simulink model "PIXELdithering_workbench"  (R2020a)
settings: Solver=FixedStepDiscrete  StartTime=0.0  StopTime=10.0  RelTol=1e-3
model workspace (MAT data in the model file):
  led0 = 1
  test = [240 320]
libraries: simulink x55, hdlsllib x29, visionsinks x2, visionzynq_privlib x2, visionhdlutilities x1, visiongeotforms x1, dspvision x1
(part 1 of 2)
settings Model: DataTypeOverride=Off  Creator=Produktivität  LastModifiedBy=Anwender
settings OptimizationCC: BlockReduction=off  ConditionallyExecuteInputs=off  DefaultParameterBehavior=Inlined
settings DebuggingCC: AlgebraicLoopMsg=error  SingleTaskRateTransMsg=error
settings HardwareCC: ProdBitPerPointer=32  ProdBitPerSizeT=32  ProdBitPerPtrDiffT=32  ProdLargestAtomicFloat=None  ProdIntDivRoundTo=Undefined  ProdEndianess=Unspecified  ProdWordSize=32  ProdHWDeviceType=ASIC/FPGA->ASIC/FPGA  TargetBitPerPointer=64  TargetBitPerSizeT=64  TargetBitPerPtrDiffT=64  TargetLongLongMode=on  TargetIntDivRoundTo=Zero  TargetEndianess=LittleEndian  TargetWordSize=64  TargetHWDeviceType=Custom Processor->MATLAB Host Computer  ProdEqTarget=off

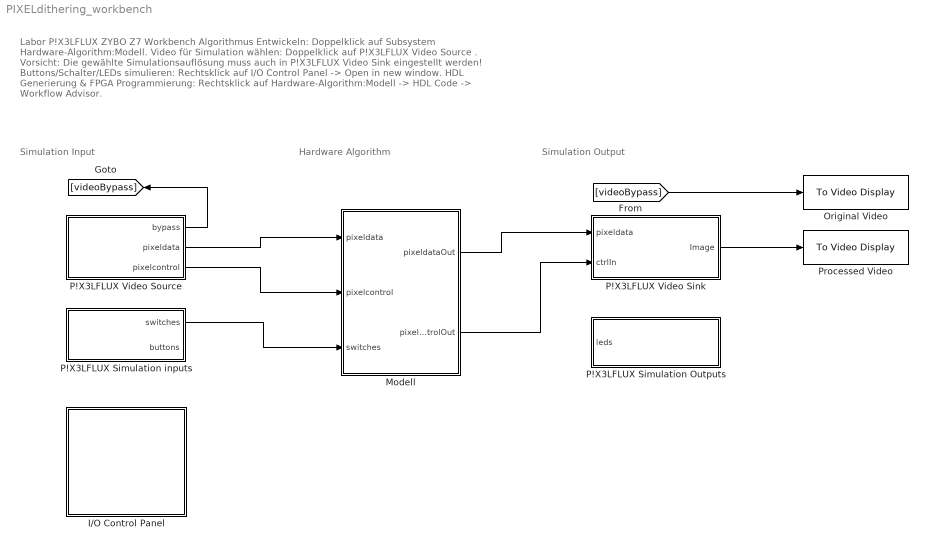
== system PIXELdithering_workbench ==
  note: Labor P!X3LFLUX
      | ZYBO Z7 Workbench
      |
      | Algorithmus Entwickeln: Doppelklick auf Subsystem Hardware-Algorithm:Modell.
      | Video für Simulation wählen: Doppelklick auf P!X3LFLUX Video Source . Vorsicht: Die gewählte Simulationsauflösung muss auch in P!X3LFLUX Video Sink eingestellt werden!
      | Buttons/Schalter/LEDs simulieren: Rechtsklick auf I/O Control Panel -> Open in new window.
      | HDL Generierung & FPGA Programmierung: Rechtsklick auf Hardware-Algorithm:Modell -> HDL Code -> Workflow Advisor.
  note: Hardware Algorithm
  note: Simulation Output
  note: Simulation Input
  I/O Control Panel : Subsystem
  Modell : Subsystem  TreatAsAtomicUnit=on
  Original Video : visionsinks/To Video Display  windowSizeMode=Normal  openAtMdlStart=on  fullScreen=off  videoWindowX=1  videoWindowY=33  saveWindowSize=off  videoWindowWidth=1916  videoWindowHeight=1006  inputColorFormat=RGB  inputType=Obsolete  imagePorts=One multidimensional signal  OutputDevice=On-screen video monitor  dataOrg=Column-major  isWindowOpen=off
  P!X3LFLUX Simulation Outputs : Subsystem
  P!X3LFLUX Simulation inputs : Subsystem  mask{buttonsMode=manual, btnFileName=mlabtest.xlsx, switchesMode=manual, swFileName=mlabtest.xlsx}
      mask prompts: buttonsMode "Buttons simulation mode:"; btnFileName "Excel filename:"; switchesMode "Switches simulation mode:"; swFileName "Excel filename:"
      mask TypeOptions buttonsMode: buttons variant choice/LabelModeActiveChoice
      mask TypeOptions btnFileName: excel reader buttons/FileName
      mask TypeOptions switchesMode: switches variant choice/LabelModeActiveChoice
      mask TypeOptions swFileName: excel reader switches/FileName
      mask DialogControl DescGroupVar Prompt: P!X3LFLUX Simulation Inputs for ZYBO Z7
      mask DialogControl DescTextVar Prompt: Dieser Block erzeugt die Simulationssignale für Knöpfe und Schalter des ZYBO Z7 Boards.
      mask DialogControl Control2 Prompt: This block generates signals for simulating the switches and buttons of the ZYBO Z7 board.
      mask DialogControl Control3 Prompt: Pick manual mode to control inputs via the I/O Control Panel
      mask DialogControl btnsContainer Prompt: Buttons simulation settings
      mask DialogControl swContainer Prompt: Switches simulation settings
  P!X3LFLUX Video Sink : Subsystem  mask{resolutionChoice=320x240}
      mask prompts: resolutionChoice "Resolution:"
      mask init:
      | resolution = get_param(gcb, 'resolutionChoice');
      | streamSinkBlk = [gcb, '/streamSink'];
      | 
      | switch resolution
      |     case '320x240'
      |         set_param(streamSinkBlk, 'FrameSize', '320x240p');
      |     case '640x480'
      |         set_param(streamSinkBlk, 'FrameSize', '640x480p');
      |     case '720x480'
      |         set_param(streamSinkBlk, 'FrameSize', '480p SDTV (720x480p)');
      |     case '1280x720'
      |         set_param(streamSinkBlk, 'FrameSize', '720p HDTV (1280x720p)');
      | end
      mask TypeOptions resolutionChoice: 320x240 | 640x480 | 720x480
      mask DialogControl DescGroupVar Prompt: P!X3LFLUX Video Sink
      mask DialogControl DescTextVar Prompt: Dieser Block wandelt einen RBG (Xilinx Encoding) Pixel Stream zurück in frames.
      mask DialogControl Control3 Prompt: This block converts a RGB (Xilinx Encoding) Pixel Stream into individual frames.
      mask DialogControl resHint Prompt: Note: Should match source resoltution!
      mask Display: image('$imagefile'); % Use "Edit Image" on toolstrip to change.
  P!X3LFLUX Video Source : Subsystem  mask{inputFilename=C:\Users\Anwender\Documents\Pixelflux_2\Boarddateien\Testdaten\360p_foggy_island.mp4, resolutionChoice=320x240}
      mask prompts: inputFilename "dspshared:FromMMFile:InputFileName"; resolutionChoice "Scaled resolution:"
      mask init:
      | resolution = get_param(gcb, 'resolutionChoice');
      | resizeBlk = [gcb, '/resizer'];
      | streamGenBlk = [gcb, '/streamGenerator'];
      | 
      | switch resolution
      |     case '320x240'
      |         set_param(streamGenBlk, 'FrameSize', '320x240p');
      |         set_param(resizeBlk, 'outRowsCols', '[240 320]');
      |     case '640x480'
      |         set_param(streamGenBlk, 'FrameSize', '640x480p');
      |         set_param(resizeBlk, 'outRowsCols', '[480 640]');
      |     case '720x480'
      |         set_param(streamGenBlk, 'FrameSize', '480p SDTV (720x480p)');
      |         set_param(resizeBlk, 'outRowsCols', '[480 720]');
      |     case '1280x720'
      |         set_param(streamGenBlk, 'FrameSize', '720p HDTV (1280x720p)');
      |         set_param(resizeBlk, 'outRowsCols', '[720 1280]');
      | end
      mask TypeOptions inputFilename: videoInput/inputFilename
      mask TypeOptions resolutionChoice: 320x240 | 640x480 | 720x480
      mask DialogControl DescGroupVar Prompt: P!X3LFLUX Lab Source
      mask DialogControl DescTextVar Prompt: Dieser Block kapselt das Einlesen eines Videofiles, Skalierung auf eine feste Auflösung sowie die Erzeugung des PixelStreams.
      mask DialogControl Control3 Prompt: This block encapsulates reading an input video file, scaling it to a fixed resolution and creating the pixel stream.
      mask DialogControl inputFilename Prompt: Input file name:
      mask DialogControl browseBtn Prompt: Browse...
      mask DialogControl browseBtn Callback:
      | [f p] = uigetfile;
      | if(f ~= 0)
      |     set_param(gcb, "inputFilename", fullfile(p, f));
      | end
      mask Display: image('$imagefile'); % Use "Edit Image" on toolstrip to change.
  Processed Video : visionsinks/To Video Display  windowSizeMode=Normal  openAtMdlStart=on  fullScreen=off  videoWindowX=1  videoWindowY=33  saveWindowSize=off  videoWindowWidth=1916  videoWindowHeight=1006  inputColorFormat=RGB  inputType=Obsolete  imagePorts=One multidimensional signal  OutputDevice=On-screen video monitor  dataOrg=Column-major  isWindowOpen=off
  wires:
  [videoBypass] -> Original Video/1
  P!X3LFLUX Video Source/1(bypass) -> [videoBypass]
  Modell/1(pixeldataOut) -> P!X3LFLUX Video Sink/1(pixeldata)
  Modell/2(pixelcontrolOut) -> P!X3LFLUX Video Sink/2(ctrlIn)
  P!X3LFLUX Video Sink/1(Image) -> Processed Video/1
  P!X3LFLUX Video Source/2(pixeldata) -> Modell/1(pixeldata)
  P!X3LFLUX Video Source/3(pixelcontrol) -> Modell/2(pixelcontrol)
  P!X3LFLUX Simulation inputs/1(switches) -> Modell/3(switches)

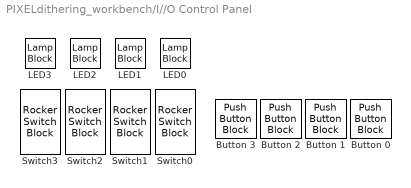
== system PIXELdithering_workbench/I//O Control Panel ==
  Button 0 : PushButtonBlock  ButtonText=0
  Button 1 : PushButtonBlock  ButtonText=1
  Button 2 : PushButtonBlock  ButtonText=2
  Button 3 : PushButtonBlock  ButtonText=3
  LED{0..3} (4 alike) : LampBlock  LabelPosition=Hide
  Switch{0..3} (4 alike) : RockerSwitchBlock  LabelPosition=Hide
      settings: Values={{'Off', 'On'}, [0 1]}

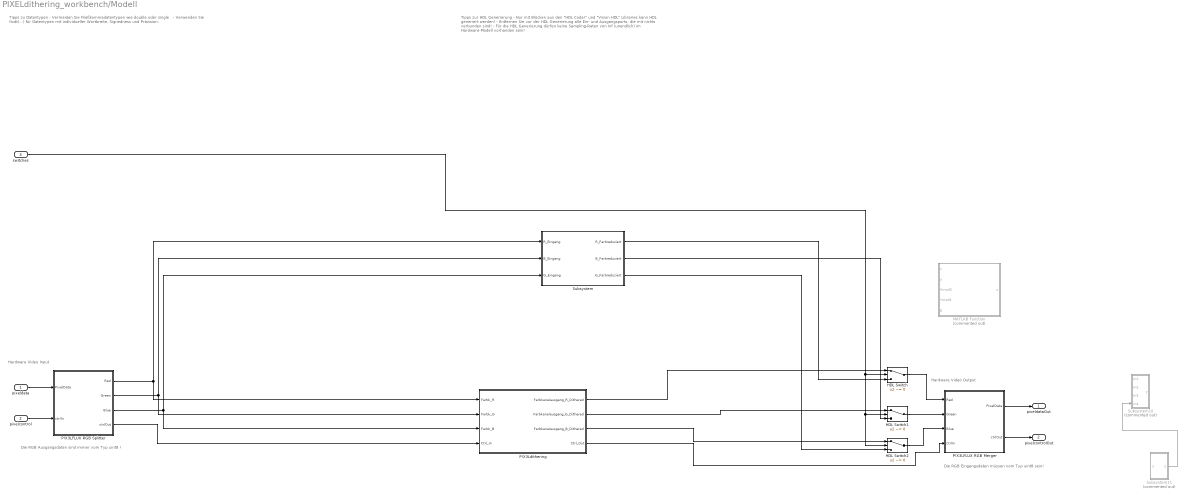
== system PIXELdithering_workbench/Modell ==
  note: Tipps zur HDL Generierung
      |
      | - Nur mit Blöcken aus den "HDL Coder" und "Vision HDL" Libraries kann HDL generiert werden!
      | - Entfernen Sie vor der HDL Generierung alle Ein- und Ausgangsports, die mit nichts verbunden sind!
      | - Für die HDL Generierung dürfen keine Sampling-Raten von Inf (unendlich) im Hardware-Modell vorhanden sein!
  note: Die RGB Ausgangsdaten sind immer vom Typ uint8 !
  note: Hardware Video Output
  note: Hardware Video Input
  note: Die RGB Eingangsdaten müssen vom Typ uint8 sein!
  note: Tipps zu Datentypen
      |
      | - Vermeiden Sie Fließkommadatentypen wie double oder single .
      | - Verwenden Sie fixdt(...) für Datentypen mit individueller Wortbreite, Signedness und Präzision.
  pixeldata : Inport  OutDataTypeStr=fixdt(0,24,0)
  pixelcontrol : Inport  Port=2  OutDataTypeStr=Bus: pixelcontrol
  switches : Inport  Port=3  OutDataTypeStr=fixdt(0,4,0)
  HDL Switch : Switch  Criteria=u2 ~= 0  Threshold=960  OutDataTypeStr=uint8
  HDL Switch1 : Switch  Criteria=u2 ~= 0  Threshold=960  OutDataTypeStr=uint8
  HDL Switch2 : Switch  Criteria=u2 ~= 0  Threshold=960  OutDataTypeStr=uint8
  MATLAB Function : MATLAB Function  Commented=on  TreatAsAtomicUnit=on
  P!X3LFLUX RGB Merger : Subsystem  Variant=on  VariantControlMode=Label  VariantControl=Choice  LabelModeActiveChoice=V_sepColor  mask{InputVersionChoice=Separate components}
      mask prompts: InputVersionChoice "Color component input mode:"
      mask init:
      | choice = get_param(gcb,'InputVersionChoice');
      | vssBlk = gcb;
      | 
      | rgbInput = find_system(gcb,...
      |     'LookUnderMasks', 'on',...
      |     'FollowLinks', 'on',...
      |     'Name', 'rgb');
      | 
      | oldVariant = get_param(gcb,'LabelModeActiveChoice');
      | if strcmp(choice,'Separate components')
      |     if ~isempty(rgbInput)
      |         delete_block([gcb, '/rgb']);
      |         add_block('built-in/Inport', [gcb, '/Red'], 'Port', '1', 'OutDataTypeStr', 'uint8', 'PortDimensions', '1');
      |         add_block('built-in/Inport', [gcb, '/Green'], 'Port', '2', 'OutDataTypeStr', 'uint8', 'PortDimensions', '1');
      |         add_block('built-in/Inport', [gcb, '/Blue'], 'Port', '3', 'OutDataTypeStr', 'uint8', 'PortDimensions', '1');
      |     end
      |     set_param(vssBlk, 'OverrideUsingVariant', 'V_sepColor');
      | else
      |     if isempty(rgbInput)
      |         delete_block([gcb, '/Red']);
      |         delete_block([gcb, '/Green']);
      |         delete_block([gcb, '/Blue']);
      |         add_block('built-in/Inport', [gcb, '/rgb'], 'Port', '1', 'OutDataTypeStr', 'uint8', 'PortDimensions', '[1 3]');
      |     end
      |     set_param(vssBlk, 'OverrideUsingVariant', 'V_vecColor');
      | end
      mask TypeOptions InputVersionChoice: Separate components | RGB vector [1x3]
      mask DialogControl DescGroupVar Prompt: P!X3LFLUX RGB Merger for Xilinx AXI4 Video Stream
      mask DialogControl DescTextVar Prompt: Dieser Block bündelt 8 Bit Farbkanäle in 24 Bit RBG (Xilinx Encoding) AXI4 Video Stream Pixeldaten. Zur HDL Generierung geeignet.
      mask DialogControl Control2 Prompt: This block packs 8 Bit color components into 24 Bit RBG (Xilinx Encoding) AXI4 Video Stream pixeldata. Compatible with HDL generation.
      mask DialogControl InputVersionChoice Tooltip: Choose between separate component ports or one [1x3] vector input
      mask Display: image('$imagefile'); % Use "Edit Image" on toolstrip to change.
  P!X3LFLUX RGB Splitter : Subsystem  Variant=on  VariantControlMode=Label  LabelModeActiveChoice=V_sepColor  mask{OutputVersionChoice=Separate components}
      mask prompts: OutputVersionChoice "Color component output mode:"
      mask init:
      | choice = get_param(gcb,'OutputVersionChoice');
      | vssBlk = gcb;
      | oldVariant = get_param(gcb,'LabelModeActiveChoice');
      | rgbOut = find_system(gcb,...
      |     'LookUnderMasks', 'on',...
      |     'FollowLinks', 'on',...
      |     'Name', 'rgb');
      | 
      | if strcmp(choice,'Separate components')
      |     if ~isempty(rgbOut)
      |         delete_block([gcb, '/rgb']);
      |         add_block('built-in/Outport', [gcb, '/Red'], 'Port', '1', 'OutDataTypeStr', 'uint8', 'PortDimensions', '1');
      |         add_block('built-in/Outport', [gcb, '/Green'], 'Port', '2', 'OutDataTypeStr', 'uint8', 'PortDimensions', '1');
      |         add_block('built-in/Outport', [gcb, '/Blue'], 'Port', '3', 'OutDataTypeStr', 'uint8', 'PortDimensions', '1');
      |     end
      |     set_param(vssBlk, 'OverrideUsingVariant', 'V_sepColor');
      | else
      |     if isempty(rgbOut)
      |         delete_block([gcb, '/Red']);
      |         delete_block([gcb, '/Green']);
      |         delete_block([gcb, '/Blue']);
      |         add_block('built-in/Outport', [gcb, '/rgb'], 'Port', '1', 'OutDataTypeStr', 'uint8', 'PortDimensions', '[1 3]');
      |     end
      |     set_param(vssBlk, 'OverrideUsingVariant', 'V_vecColor');
      | end
      mask TypeOptions OutputVersionChoice: Separate components | RGB vector [1x3]
      mask DialogControl DescGroupVar Prompt: P!X3LFLUX RGB Splitter for Xilinx AXI4 Video Stream
      mask DialogControl DescGerman Prompt: Dieser Block separiert die Farbkanäle von 24 Bit RBG (Xilinx Encoding) AXI4 Video Stream Pixeldaten.
      mask DialogControl DescEnglish Prompt: This block separates the color components of 24 Bit RBG (Xilinx Encoding) AXI4 Video Stream pixel data.
      mask Display: image('$imagefile'); % Use "Edit Image" on toolstrip to change.
  P!X3Ldithering : Subsystem
  Subsystem : Subsystem
  Subsystem10 : Subsystem  Commented=on
  Subsystem11 : Subsystem  Commented=on
  pixeldataOut : Outport  OutDataTypeStr=fixdt(0,24,0)  VectorParamsAs1DForOutWhenUnconnected=off
  pixelcontrolOut : Outport  Port=2  VectorParamsAs1DForOutWhenUnconnected=off
  wires:
  P!X3LFLUX RGB Merger/1(PixelData) -> pixeldataOut/1
  P!X3LFLUX RGB Merger/2(ctrlOut) -> pixelcontrolOut/1
  pixeldata/1 -> P!X3LFLUX RGB Splitter/1(PixelData)
  pixelcontrol/1 -> P!X3LFLUX RGB Splitter/2(ctrlIn)
  HDL Switch/1 -> P!X3LFLUX RGB Merger/1(Red)
  HDL Switch1/1 -> P!X3LFLUX RGB Merger/2(Green)
  HDL Switch2/1 -> P!X3LFLUX RGB Merger/3(Blue)
  switches/1 -> HDL Switch2/2, HDL Switch1/2, HDL Switch/2
  Subsystem11/1(Out1) -> Subsystem10/4(In4)
  Subsystem/1(R_Farbreduziert) -> HDL Switch/3
  Subsystem/2(B_Farbreduziert) -> HDL Switch1/3
  Subsystem/3(G_Farbreduziert) -> HDL Switch2/3
  P!X3LFLUX RGB Splitter/1(Red) -> Subsystem/1(R_Eingang), P!X3Ldithering/1(Farbk_R)
  P!X3LFLUX RGB Splitter/2(Green) -> Subsystem/2(B_Eingang), P!X3Ldithering/2(Farbk_G)
  P!X3LFLUX RGB Splitter/3(Blue) -> Subsystem/3(G_Eingang), P!X3Ldithering/3(Farbk_B)
  P!X3LFLUX RGB Splitter/4(ctrlOut) -> P!X3Ldithering/4(Ctrl_In)
  P!X3Ldithering/1(Farbkanalausgang_R_Dithered) -> HDL Switch/1
  P!X3Ldithering/2(Farbkanalausgang_G_Dithered) -> HDL Switch1/1
  P!X3Ldithering/3(Farbkanalausgang_B_Dithered) -> HDL Switch2/1
  P!X3Ldithering/4(Ctrl_Out) -> P!X3LFLUX RGB Merger/4(ctrlIn)

== system PIXELdithering_workbench/P!X3LFLUX Simulation Outputs ==
  leds : Inport  OutDataTypeStr=fixdt(0,4,0)
  Display{,1..3} (4 alike) : Display
  Extract Bits : simulink/Logic and Bit Operations/Extract Bits  bitsToExtract=Range of bits  numBits=8  bitIdxRange=[0 0]  outScalingMode=Treat bit field as an integer
  Extract Bits1 : simulink/Logic and Bit Operations/Extract Bits  bitsToExtract=Range of bits  numBits=8  bitIdxRange=[1 1]  outScalingMode=Treat bit field as an integer
  Extract Bits2 : simulink/Logic and Bit Operations/Extract Bits  bitsToExtract=Range of bits  numBits=8  bitIdxRange=[2 2]  outScalingMode=Treat bit field as an integer
  Extract Bits3 : simulink/Logic and Bit Operations/Extract Bits  bitsToExtract=Range of bits  numBits=8  bitIdxRange=[3 3]  outScalingMode=Treat bit field as an integer
  wires:
  leds/1 -> Extract Bits/1, Extract Bits1/1, Extract Bits3/1, Extract Bits2/1
  Extract Bits1/1 -> Display1/1
  Extract Bits2/1 -> Display2/1
  Extract Bits3/1 -> Display3/1
  Extract Bits/1 -> Display/1

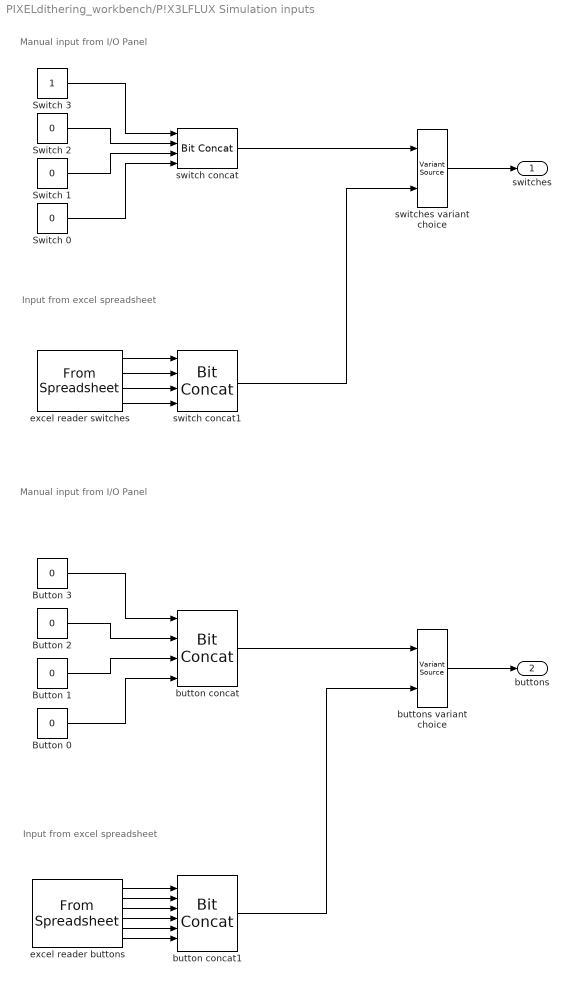
== system PIXELdithering_workbench/P!X3LFLUX Simulation inputs ==
  note: Input from excel spreadsheet
  note: Manual input from I/O Panel
  note: Manual input from I/O Panel
  note: Input from excel spreadsheet
  Button {0..3} (4 alike) : Constant  Value=0  OutDataTypeStr=boolean
  Switch 0 : Constant  Value=0  OutDataTypeStr=boolean
  Switch 1 : Constant  Value=0  OutDataTypeStr=boolean
  Switch 2 : Constant  Value=0  OutDataTypeStr=boolean
  Switch 3 : Constant  OutDataTypeStr=boolean
  button concat : hdlsllib/Logic and Bit Operations/Bit Concat  numInputs=4
  button concat1 : hdlsllib/Logic and Bit Operations/Bit Concat  numInputs=6
  buttons variant choice : VariantSource  VariantControlMode=Label  LabelModeActiveChoice=manual
  excel reader buttons : FromSpreadsheet  FileName=mlabtest.xlsx  SheetName=buttons  OutDataTypeStr=boolean  ExtrapolationBeforeFirstDataPoint=Ground value  InterpolationWithinTimeRange=Zero order hold  ExtrapolationAfterLastDataPoint=Hold last value
  excel reader switches : FromSpreadsheet  FileName=mlabtest.xlsx  SheetName=switches  OutDataTypeStr=boolean  ExtrapolationBeforeFirstDataPoint=Ground value  InterpolationWithinTimeRange=Zero order hold  ExtrapolationAfterLastDataPoint=Hold last value
  switch concat : hdlsllib/Logic and Bit Operations/Bit Concat  numInputs=4
  switch concat1 : hdlsllib/Logic and Bit Operations/Bit Concat  numInputs=4
  switches variant choice : VariantSource  VariantControlMode=Label  LabelModeActiveChoice=manual
  switches : Outport  OutDataTypeStr=fixdt(0,4,0)
  buttons : Outport  Port=2  OutDataTypeStr=fixdt(0,4,0)
  wires:
  Switch 3/1 -> switch concat/1
  Switch 2/1 -> switch concat/2
  Switch 1/1 -> switch concat/3
  Switch 0/1 -> switch concat/4
  switch concat/1 -> switches variant choice/1
  excel reader buttons/6 -> button concat1/6
  excel reader buttons/5 -> button concat1/5
  excel reader buttons/4 -> button concat1/4
  excel reader buttons/3 -> button concat1/3
  excel reader buttons/2 -> button concat1/2
  excel reader buttons/1 -> button concat1/1
  excel reader switches/1 -> switch concat1/1
  excel reader switches/2 -> switch concat1/2
  excel reader switches/3 -> switch concat1/3
  excel reader switches/4 -> switch concat1/4
  switch concat1/1 -> switches variant choice/2
  button concat1/1 -> buttons variant choice/2
  switches variant choice/1 -> switches/1
  button concat/1 -> buttons variant choice/1
  buttons variant choice/1 -> buttons/1
  Button 3/1 -> button concat/1
  Button 2/1 -> button concat/2
  Button 1/1 -> button concat/3
  Button 0/1 -> button concat/4

== system PIXELdithering_workbench/P!X3LFLUX Video Sink ==
  pixeldata : Inport
  ctrlIn : Inport  Port=2
  Terminator : Terminator
  Xilinx2RGB : Subsystem
  streamSink : visionzynq_privlib/Image Pixels To Frame  FrameSize=320x240p
      settings: SourceProductBaseCode=VP_VISION_ZYNQ
  Image : Outport
  wires:
  ctrlIn/1 -> Xilinx2RGB/2(ctrlIn)
  Xilinx2RGB/1(rgbVector) -> streamSink/1
  Xilinx2RGB/2(ctrlOut) -> streamSink/2
  pixeldata/1 -> Xilinx2RGB/1(rbgXilinx)
  streamSink/1 -> Image/1
  streamSink/2 -> Terminator/1

== system PIXELdithering_workbench/P!X3LFLUX Video Source ==
  RGB2Xilinx : Subsystem
  resizer : visiongeotforms/Resize  specify=Number of output rows and columns  rfactor=[200 150]  outCols=320  outRows=25  outRowsCols=[240 320]  interp_method=Bilinear  antialias=on  useROI=off  roiFlag=off  roundingMode=Nearest  overflowMode=on  prodOutputMode=Binary point scaling  prodOutputWordLength=32  prodOutputFracLength=10
      settings: SourceProductBaseCode=VP
  streamGenerator : visionzynq_privlib/Image Frame To Pixels   FrameSize=320x240p
      settings: SourceProductBaseCode=VP_VISION_ZYNQ
  videoInput : dspvision/From Multimedia File  inputFilename=C:\Users\Anwender\Documents\Pixelflux_2\Boarddateien\Testdaten\360p_foggy_island.mp4  readRange=[1 Inf]  loop=on  numPlays=inf  outputStreams=Video only  videoDataType=uint8  audioDataType=int16  inheritSampleTime=on  userDefinedSampleTime=1/30  noAudioOutput=off  isIntensityVideo=off  fourcc=RGB  colorVideoFormat=One multidimensional signal  outputEOF=off  dataOrg=Column-major  audioFrameSize=1024  computeAudioFrameSize=off  outSamplingMode=Sample based
  bypass : Outport
  pixeldata : Outport  Port=2
  pixelcontrol : Outport  Port=3
  wires:
  streamGenerator/1 -> RGB2Xilinx/1(rgbVector)
  resizer/1 -> bypass/1, streamGenerator/1
  videoInput/1 -> resizer/1
  streamGenerator/2 -> RGB2Xilinx/2(ctrlIn)
  RGB2Xilinx/1(rbgXilinx) -> pixeldata/1
  RGB2Xilinx/2(ctrlOut) -> pixelcontrol/1

== system PIXELdithering_workbench/Modell/P!X3LFLUX RGB Merger ==
  Red : Inport  OutDataTypeStr=uint8  PortDimensions=1
  Green : Inport  Port=2  OutDataTypeStr=uint8  PortDimensions=1
  Blue : Inport  Port=3  OutDataTypeStr=uint8  PortDimensions=1
  ctrlIn : Inport  Port=4  OutDataTypeStr=Bus: pixelcontrol
  scalar mode : Subsystem  VariantControl=V_sepColor
  vector mode : Subsystem  VariantControl=V_vecColor
  PixelData : Outport  OutDataTypeStr=fixdt(0,24,0)
  ctrlOut : Outport  Port=2  OutDataTypeStr=Bus: pixelcontrol

== system PIXELdithering_workbench/Modell/P!X3LFLUX RGB Splitter ==
  PixelData : Inport
  ctrlIn : Inport  Port=2  OutDataTypeStr=Bus: pixelcontrol
  " vector mode" : Subsystem  VariantControl=V_vecColor
  scalar mode : Subsystem  VariantControl=V_sepColor
  Red : Outport  OutDataTypeStr=uint8  PortDimensions=1
  Green : Outport  Port=2  OutDataTypeStr=uint8  PortDimensions=1
  Blue : Outport  Port=3  OutDataTypeStr=uint8  PortDimensions=1
  ctrlOut : Outport  Port=4  VectorParamsAs1DForOutWhenUnconnected=off

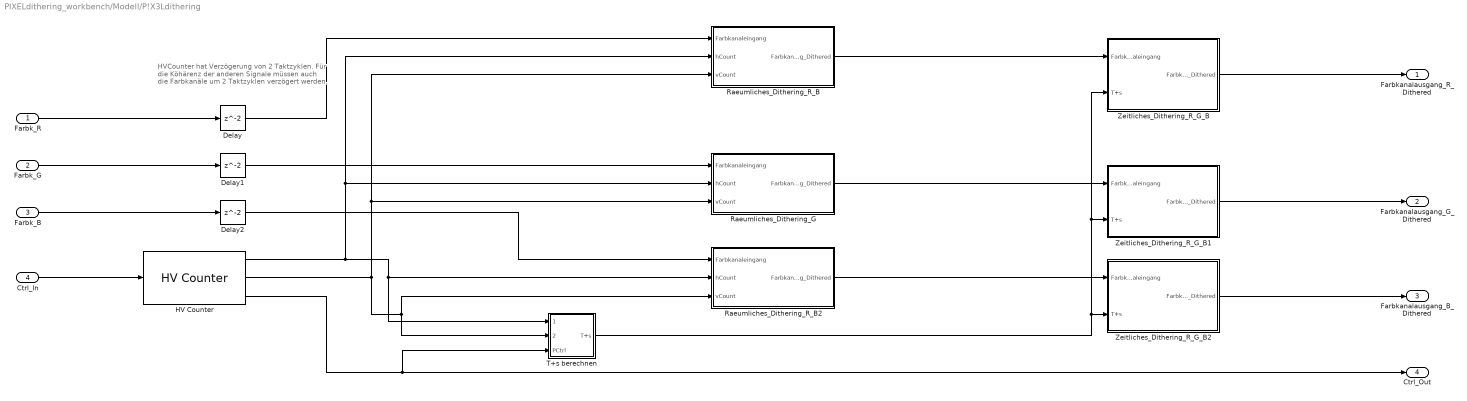
== system PIXELdithering_workbench/Modell/P!X3Ldithering ==
  note: HVCounter hat Verzögerung von 2 Taktzyklen.
      | Für die Köhärenz der anderen Signale müssen
      | auch die Farbkanäle um 2 Taktzyklen verzögert
      | werden.
  Farbk_R : Inport
  Farbk_G : Inport  Port=2
  Farbk_B : Inport  Port=3
  Ctrl_In : Inport  Port=4
  Delay : Delay  InitialCondition=0
  Delay1 : Delay  InitialCondition=0
  Delay2 : Delay  InitialCondition=0
  HV Counter : visionhdlutilities/HV Counter  ActivePixelsPerLine=1920  ActiveVideoLines=1080  SimulateUsing=Code generation
      settings: SourceProductBaseCode=VT
  Raeumliches_Dithering_G : Subsystem
  Raeumliches_Dithering_R_B : Subsystem
  Raeumliches_Dithering_R_B2 : Subsystem
  T+s berechnen : Subsystem
  Zeitliches_Dithering_R_G_B : Subsystem
  Zeitliches_Dithering_R_G_B1 : Subsystem
  Zeitliches_Dithering_R_G_B2 : Subsystem
  Farbkanalausgang_R_Dithered : Outport
  Farbkanalausgang_G_Dithered : Outport  Port=2
  Farbkanalausgang_B_Dithered : Outport  Port=3
  Ctrl_Out : Outport  Port=4
  wires:
  Zeitliches_Dithering_R_G_B2/1(Farbkanalausgang_Dithered) -> Farbkanalausgang_B_Dithered/1
  Farbk_G/1 -> Delay1/1
  HV Counter/1 -> T+s berechnen/1(hCount), Raeumliches_Dithering_R_B2/2(hCount), Raeumliches_Dithering_G/2(hCount), Raeumliches_Dithering_R_B/2(hCount)
  Farbk_B/1 -> Delay2/1
  T+s berechnen/1(T+s) -> Zeitliches_Dithering_R_G_B2/2(T+s), Zeitliches_Dithering_R_G_B1/2(T+s), Zeitliches_Dithering_R_G_B/2(T+s)
  HV Counter/2 -> Raeumliches_Dithering_R_B2/3(vCount), T+s berechnen/2(vCount), Raeumliches_Dithering_G/3(vCount), Raeumliches_Dithering_R_B/3(vCount)
  Delay2/1 -> Raeumliches_Dithering_R_B2/1(Farbkanaleingang)
  HV Counter/3 -> Ctrl_Out/1, T+s berechnen/3(PCtrl)
  Zeitliches_Dithering_R_G_B/1(Farbkanalausgang_Dithered) -> Farbkanalausgang_R_Dithered/1
  Raeumliches_Dithering_G/1(Farbkanalausgang_Dithered) -> Zeitliches_Dithering_R_G_B1/1(Farbkanaleingang)
  Delay/1 -> Raeumliches_Dithering_R_B/1(Farbkanaleingang)
  Raeumliches_Dithering_R_B/1(Farbkanalausgang_Dithered) -> Zeitliches_Dithering_R_G_B/1(Farbkanaleingang)
  Delay1/1 -> Raeumliches_Dithering_G/1(Farbkanaleingang)
  Raeumliches_Dithering_R_B2/1(Farbkanalausgang_Dithered) -> Zeitliches_Dithering_R_G_B2/1(Farbkanaleingang)
  Ctrl_In/1 -> HV Counter/1
  Zeitliches_Dithering_R_G_B1/1(Farbkanalausgang_Dithered) -> Farbkanalausgang_G_Dithered/1
  Farbk_R/1 -> Delay/1

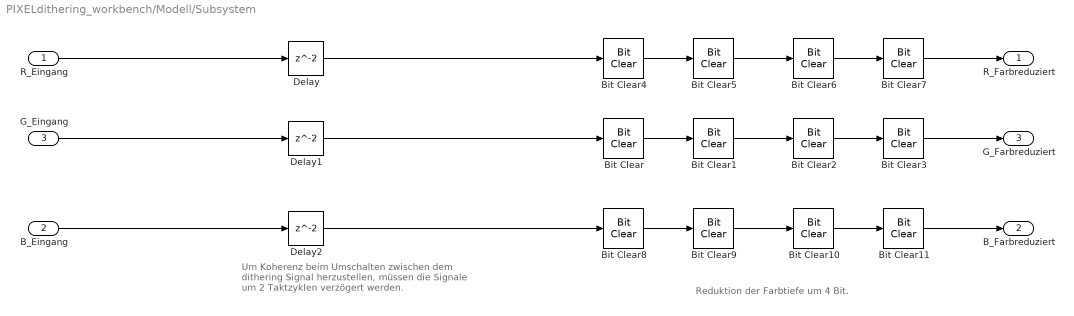
== system PIXELdithering_workbench/Modell/Subsystem ==
  note: Um Koherenz beim Umschalten zwischen dem
      | dithering Signal herzustellen, müssen die
      | Signale um 2 Taktzyklen verzögert werden.
  note: Reduktion der Farbtiefe um 4 Bit.
  R_Eingang : Inport
  B_Eingang : Inport  Port=2
  G_Eingang : Inport  Port=3
  Bit Clear : simulink/Logic and Bit Operations/Bit Clear  iBit=0
      settings: SourceProductBaseCode=SL
  Bit Clear1 : simulink/Logic and Bit Operations/Bit Clear  iBit=1
      settings: SourceProductBaseCode=SL
  Bit Clear10 : simulink/Logic and Bit Operations/Bit Clear  iBit=2
      settings: SourceProductBaseCode=SL
  Bit Clear11 : simulink/Logic and Bit Operations/Bit Clear  iBit=3
      settings: SourceProductBaseCode=SL
  Bit Clear2 : simulink/Logic and Bit Operations/Bit Clear  iBit=2
      settings: SourceProductBaseCode=SL
  Bit Clear3 : simulink/Logic and Bit Operations/Bit Clear  iBit=3
      settings: SourceProductBaseCode=SL
  Bit Clear4 : simulink/Logic and Bit Operations/Bit Clear  iBit=0
      settings: SourceProductBaseCode=SL
  Bit Clear5 : simulink/Logic and Bit Operations/Bit Clear  iBit=1
      settings: SourceProductBaseCode=SL
  Bit Clear6 : simulink/Logic and Bit Operations/Bit Clear  iBit=2
      settings: SourceProductBaseCode=SL
  Bit Clear7 : simulink/Logic and Bit Operations/Bit Clear  iBit=3
      settings: SourceProductBaseCode=SL
  Bit Clear8 : simulink/Logic and Bit Operations/Bit Clear  iBit=0
      settings: SourceProductBaseCode=SL
  Bit Clear9 : simulink/Logic and Bit Operations/Bit Clear  iBit=1
      settings: SourceProductBaseCode=SL
  Delay : Delay  InitialCondition=0
  Delay1 : Delay  InitialCondition=0
  Delay2 : Delay  InitialCondition=0
  R_Farbreduziert : Outport
  B_Farbreduziert : Outport  Port=2
  G_Farbreduziert : Outport  Port=3
  wires:
  Bit Clear4/1 -> Bit Clear5/1
  Bit Clear10/1 -> Bit Clear11/1
  Bit Clear/1 -> Bit Clear1/1
  Bit Clear1/1 -> Bit Clear2/1
  Bit Clear9/1 -> Bit Clear10/1
  Bit Clear5/1 -> Bit Clear6/1
  Bit Clear3/1 -> G_Farbreduziert/1
  Bit Clear2/1 -> Bit Clear3/1
  Bit Clear8/1 -> Bit Clear9/1
  Bit Clear6/1 -> Bit Clear7/1
  Bit Clear7/1 -> R_Farbreduziert/1
  Bit Clear11/1 -> B_Farbreduziert/1
  R_Eingang/1 -> Delay/1
  Delay/1 -> Bit Clear4/1
  G_Eingang/1 -> Delay1/1
  Delay1/1 -> Bit Clear/1
  B_Eingang/1 -> Delay2/1
  Delay2/1 -> Bit Clear8/1

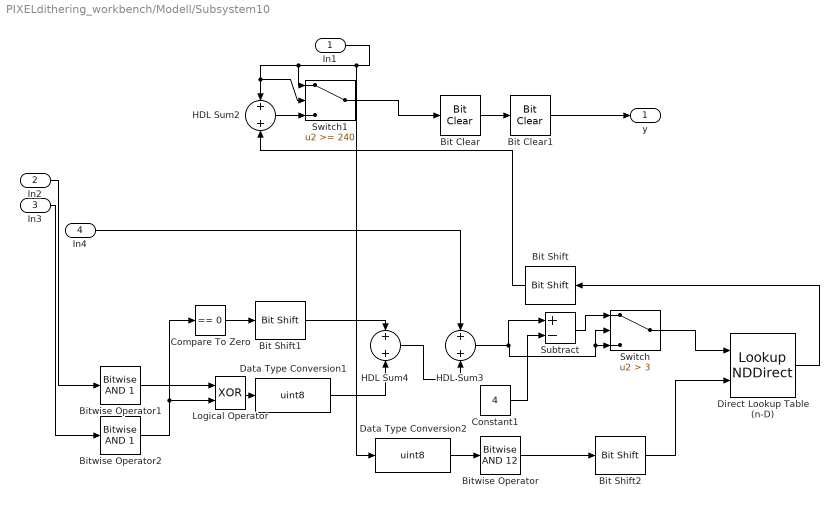
== system PIXELdithering_workbench/Modell/Subsystem10 ==
  In1 : Inport
  In2 : Inport  Port=2
  In3 : Inport  Port=3
  In4 : Inport  Port=4
  Bit Clear : simulink/Logic and Bit Operations/Bit Clear  iBit=2
      settings: SourceProductBaseCode=SL
  Bit Clear1 : simulink/Logic and Bit Operations/Bit Clear  iBit=3
      settings: SourceProductBaseCode=SL
  Bit Shift : hdlsllib/Logic and Bit Operations/Bit Shift  mode=Shift Left Logical  N=4
  Bit Shift1 : hdlsllib/Logic and Bit Operations/Bit Shift  mode=Shift Left Logical  N=1
  Bit Shift2 : hdlsllib/Logic and Bit Operations/Bit Shift  mode=Shift Right Logical  N=2
  Bitwise Operator : simulink/Logic and Bit Operations/Bitwise Operator  logicop=AND  UseBitMask=on  BitMask=12  BitMaskRealWorld=Stored Integer
  Bitwise Operator1 : simulink/Logic and Bit Operations/Bitwise Operator  logicop=AND  UseBitMask=on  BitMask=1  BitMaskRealWorld=Stored Integer
  Bitwise Operator2 : simulink/Logic and Bit Operations/Bitwise Operator  logicop=AND  UseBitMask=on  BitMask=1  BitMaskRealWorld=Stored Integer
  Compare To Zero : simulink/Logic and Bit Operations/Compare To Zero  relop===  OutDataTypeStr=uint8
  Constant1 : Constant  Value=4  OutDataTypeStr=uint8  SampleTime=-1
  Data Type Conversion1 : DataTypeConversion  OutMin=0  OutMax=1  OutDataTypeStr=uint8
  Data Type Conversion2 : DataTypeConversion  OutDataTypeStr=uint8
  Direct Lookup Table (n-D) : LookupNDDirect  Table=[0 1 1 0; 0 0 0 1; 0 0 1 1; 0 0 0 1]  DiagnosticForOutOfRangeInput=Error  TableDataTypeStr=uint8
  HDL Sum2 : Sum  OutDataTypeStr=uint8  SaturateOnIntegerOverflow=on
  HDL Sum3 : Sum  OutDataTypeStr=uint8  SaturateOnIntegerOverflow=on
  HDL Sum4 : Sum  OutDataTypeStr=uint8  SaturateOnIntegerOverflow=on
  Logical Operator : Logic  Operator=XOR  AllPortsSameDT=off  OutDataTypeStr=fixdt(1,16)
  Subtract : Sum  Inputs=+-
  Switch : Switch  Criteria=u2 > Threshold  Threshold=3
  Switch1 : Switch  Threshold=240
  y : Outport
  wires:
  Bitwise Operator1/1 -> Logical Operator/1
  Direct Lookup Table (n-D)/1 -> Bit Shift/1
  Bit Shift/1 -> HDL Sum2/2
  In1/1 -> Switch1/1, Switch1/2, HDL Sum2/1, Data Type Conversion2/1
  Constant1/1 -> Subtract/2
  Bit Clear/1 -> Bit Clear1/1
  Switch/1 -> Direct Lookup Table (n-D)/1
  HDL Sum3/1 -> Subtract/1, Switch/3, Switch/2
  Bitwise Operator2/1 -> Compare To Zero/1, Logical Operator/2
  Data Type Conversion1/1 -> HDL Sum4/2
  Bit Shift1/1 -> HDL Sum4/1
  Compare To Zero/1 -> Bit Shift1/1
  HDL Sum4/1 -> HDL Sum3/2
  Logical Operator/1 -> Data Type Conversion1/1
  Bit Clear1/1 -> y/1
  Subtract/1 -> Switch/1
  In2/1 -> Bitwise Operator1/1
  In3/1 -> Bitwise Operator2/1
  Bitwise Operator/1 -> Bit Shift2/1
  Bit Shift2/1 -> Direct Lookup Table (n-D)/2
  Data Type Conversion2/1 -> Bitwise Operator/1
  HDL Sum2/1 -> Switch1/3
  Switch1/1 -> Bit Clear/1
  In4/1 -> HDL Sum3/1

== system PIXELdithering_workbench/Modell/Subsystem11 ==
  In1 : Inport
  Bus Selector : BusSelector  OutputSignals=vEnd
  Constant : Constant  Value=0  OutDataTypeStr=uint8  SampleTime=-1
  Data Type Conversion : DataTypeConversion  OutMin=0  OutMax=1  OutDataTypeStr=uint8
  HDL Sum1 : Sum  OutDataTypeStr=uint8  SaturateOnIntegerOverflow=on
  HDL Switch3 : Switch  Criteria=u2 > Threshold  Threshold=3  OutDataTypeStr=uint8
  Memory : Memory  InheritSampleTime=on
  Out1 : Outport
  wires:
  HDL Switch3/1 -> Out1/1, Memory/1
  Data Type Conversion/1 -> HDL Sum1/1
  Constant/1 -> HDL Switch3/1
  HDL Sum1/1 -> HDL Switch3/2, HDL Switch3/3
  Memory/1 -> HDL Sum1/2
  Bus Selector/1 -> Data Type Conversion/1  "<vEnd>"
  In1/1 -> Bus Selector/1

== system PIXELdithering_workbench/P!X3LFLUX Video Sink/Xilinx2RGB ==
  note: RBG2RGB Kurzbeschreibung/brief description
      |
      | Deutsch
      | Dieser Block wandelt die bei Xilinx AXI4 Video Stream IPs verwendete RBG (B/G getauscht) Codierung in das Matlab RGB Vektor-Format (uint8 [1x3] shape).
      | Für die einfache Adaption an DUTs in der Simulation.
      | (Für nähere Informationen zum Xilinx Encoding siehe Xilinx Dokument UG934 S. 8ff, Version vom 30.10.2019)
      |
      | English
      | This block converts the RBG (B/G flipped) packed encoding used in Xilinx AXI4 Video Streams into the usual Matlab RGB vector format (uint8 [1x3] shape).
      | Allows for easy adaptation in simulations.
  rbgXilinx : Inport  OutDataTypeStr=fixdt(0,24,0)  PortDimensions=1
  ctrlIn : Inport  Port=2
  Bit Slice : hdlsllib/Logic and Bit Operations/Bit Slice  lidx=23  ridx=16
      settings: SourceProductBaseCode=SL
  Bit Slice1 : hdlsllib/Logic and Bit Operations/Bit Slice  lidx=7  ridx=0
      settings: SourceProductBaseCode=SL
  Bit Slice2 : hdlsllib/Logic and Bit Operations/Bit Slice  lidx=15  ridx=8
      settings: SourceProductBaseCode=SL
  Vector Concatenate : Concatenate  NumInputs=3  Mode=Multidimensional array  ConcatenateDimension=2
  rgbVector : Outport  OutDataTypeStr=uint8  PortDimensions=[1 3]
  ctrlOut : Outport  Port=2
  wires:
  rbgXilinx/1 -> Bit Slice/1, Bit Slice2/1, Bit Slice1/1  "Xilinx Encoding (RBG)"
  Bit Slice/1 -> Vector Concatenate/1  "Red"
  Bit Slice1/1 -> Vector Concatenate/2  "Green"
  Bit Slice2/1 -> Vector Concatenate/3  "Blue"
  Vector Concatenate/1 -> rgbVector/1  "RGB Vector"
  ctrlIn/1 -> ctrlOut/1  "pixelcontrol passthrough"

== system PIXELdithering_workbench/P!X3LFLUX Video Source/RGB2Xilinx ==
  note: RGB2Xilinx Kurzbeschreibung/brief description
      |
      | Deutsch
      | Dieser Block wandelt das Matlab RGB Vektor-Format (uint8 [1x3] shape) in die bei Xilinx AXI4 Video Stream IPs verwendete RBG (B/G getauscht) Codierung.
      | Für die einfache Adaption an DUTs in der Simulation.
      | (Für nähere Informationen zum Xilinx Encoding siehe Xilinx Dokument UG934 S. 8ff, Version vom 30.10.2019)
      |
      | English
      | This block converts the usual Matlab RGB vector format (uint8 [1x3] shape) into the RBG (B/G flipped) packed encoding used in Xilinx AXI4 Video Streams.
      | Allows for easy adaptation in simulations.
  rgbVector : Inport  OutDataTypeStr=uint8  PortDimensions=[1 3]
  ctrlIn : Inport  Port=2
  Bit Concat : hdlsllib/Logic and Bit Operations/Bit Concat  numInputs=3
  Select Blue : Selector  NumberOfDimensions=2  InputPortWidth=3  IndexOptions=Select all,Index vector (dialog)  Indices=[1 3],3  OutputSizes=1,1
  Select Green : Selector  NumberOfDimensions=2  InputPortWidth=3  IndexOptions=Select all,Index vector (dialog)  Indices=[1 3],2  OutputSizes=1,1
  Select Red : Selector  NumberOfDimensions=2  InputPortWidth=3  IndexOptions=Select all,Index vector (dialog)  Indices=[1 3],1  OutputSizes=1,1
  rbgXilinx : Outport
  ctrlOut : Outport  Port=2
  wires:
  rgbVector/1 -> Select Green/1, Select Blue/1, Select Red/1  "RGB vector"
  Bit Concat/1 -> rbgXilinx/1  "Xilinx Encoding (RBG)"
  Select Red/1 -> Bit Concat/1  "Red"
  Select Blue/1 -> Bit Concat/2  "Blue"
  Select Green/1 -> Bit Concat/3  "Green"
  ctrlIn/1 -> ctrlOut/1

== system PIXELdithering_workbench/Modell/P!X3LFLUX RGB Merger/scalar mode ==
  Red : Inport  OutDataTypeStr=uint8
  Green : Inport  Port=2  OutDataTypeStr=uint8
  Blue : Inport  Port=3  OutDataTypeStr=uint8
  ctrlIn : Inport  Port=4  OutDataTypeStr=Bus: pixelcontrol
  Bit Concat : hdlsllib/Logic and Bit Operations/Bit Concat  numInputs=3
  PixelData : Outport  OutDataTypeStr=fixdt(0,24,0)  VectorParamsAs1DForOutWhenUnconnected=off
  ctrlOut : Outport  Port=2  VectorParamsAs1DForOutWhenUnconnected=off
  wires:
  ctrlIn/1 -> ctrlOut/1
  Bit Concat/1 -> PixelData/1
  Red/1 -> Bit Concat/1
  Blue/1 -> Bit Concat/2
  Green/1 -> Bit Concat/3

== system PIXELdithering_workbench/Modell/P!X3LFLUX RGB Merger/vector mode ==
  rgb : Inport  OutDataTypeStr=uint8  PortDimensions=[1 3]
  ctrlIn : Inport  Port=2  OutDataTypeStr=Bus: pixelcontrol
  Bit Concat : hdlsllib/Logic and Bit Operations/Bit Concat  numInputs=3
  Demux : Demux  Outputs=3
  PixelData : Outport  OutDataTypeStr=fixdt(0,24,0)  VectorParamsAs1DForOutWhenUnconnected=off
  ctrlOut : Outport  Port=2  VectorParamsAs1DForOutWhenUnconnected=off
  wires:
  ctrlIn/1 -> ctrlOut/1
  Bit Concat/1 -> PixelData/1
  Demux/1 -> Bit Concat/1
  Demux/3 -> Bit Concat/2
  rgb/1 -> Demux/1
  Demux/2 -> Bit Concat/3

== system PIXELdithering_workbench/Modell/P!X3LFLUX RGB Splitter/ vector mode ==
  PixelData : Inport  OutDataTypeStr=fixdt(0,24,0)
  ctrlIn : Inport  Port=2  OutDataTypeStr=Bus: pixelcontrol
  Bit Slice : hdlsllib/Logic and Bit Operations/Bit Slice  lidx=23  ridx=16
      settings: SourceProductBaseCode=SL
  Bit Slice1 : hdlsllib/Logic and Bit Operations/Bit Slice  lidx=7  ridx=0
      settings: SourceProductBaseCode=SL
  Bit Slice2 : hdlsllib/Logic and Bit Operations/Bit Slice  lidx=15  ridx=8
      settings: SourceProductBaseCode=SL
  Vector Concatenate : Concatenate  NumInputs=3  Mode=Multidimensional array  ConcatenateDimension=2
  rgb : Outport  OutDataTypeStr=uint8  PortDimensions=[1 3]  VectorParamsAs1DForOutWhenUnconnected=off
  ctrlOut : Outport  Port=2  VectorParamsAs1DForOutWhenUnconnected=off
  wires:
  PixelData/1 -> Bit Slice2/1, Bit Slice1/1, Bit Slice/1
  Bit Slice1/1 -> Vector Concatenate/2
  Bit Slice/1 -> Vector Concatenate/1
  Bit Slice2/1 -> Vector Concatenate/3
  Vector Concatenate/1 -> rgb/1
  ctrlIn/1 -> ctrlOut/1

== system PIXELdithering_workbench/Modell/P!X3LFLUX RGB Splitter/scalar mode ==
  PixelData : Inport  OutDataTypeStr=fixdt(0,24,0)
  ctrlIn : Inport  Port=2  OutDataTypeStr=Bus: pixelcontrol
  Bit Slice : hdlsllib/Logic and Bit Operations/Bit Slice  lidx=23  ridx=16
      settings: SourceProductBaseCode=SL
  Bit Slice1 : hdlsllib/Logic and Bit Operations/Bit Slice  lidx=7  ridx=0
      settings: SourceProductBaseCode=SL
  Bit Slice2 : hdlsllib/Logic and Bit Operations/Bit Slice  lidx=15  ridx=8
      settings: SourceProductBaseCode=SL
  Red : Outport  OutDataTypeStr=uint8  VectorParamsAs1DForOutWhenUnconnected=off
  Green : Outport  Port=2  OutDataTypeStr=uint8  VectorParamsAs1DForOutWhenUnconnected=off
  Blue : Outport  Port=3  OutDataTypeStr=uint8  VectorParamsAs1DForOutWhenUnconnected=off
  ctrlOut : Outport  Port=4  VectorParamsAs1DForOutWhenUnconnected=off
  wires:
  PixelData/1 -> Bit Slice2/1, Bit Slice1/1, Bit Slice/1
  Bit Slice1/1 -> Green/1
  Bit Slice/1 -> Red/1
  Bit Slice2/1 -> Blue/1
  ctrlIn/1 -> ctrlOut/1

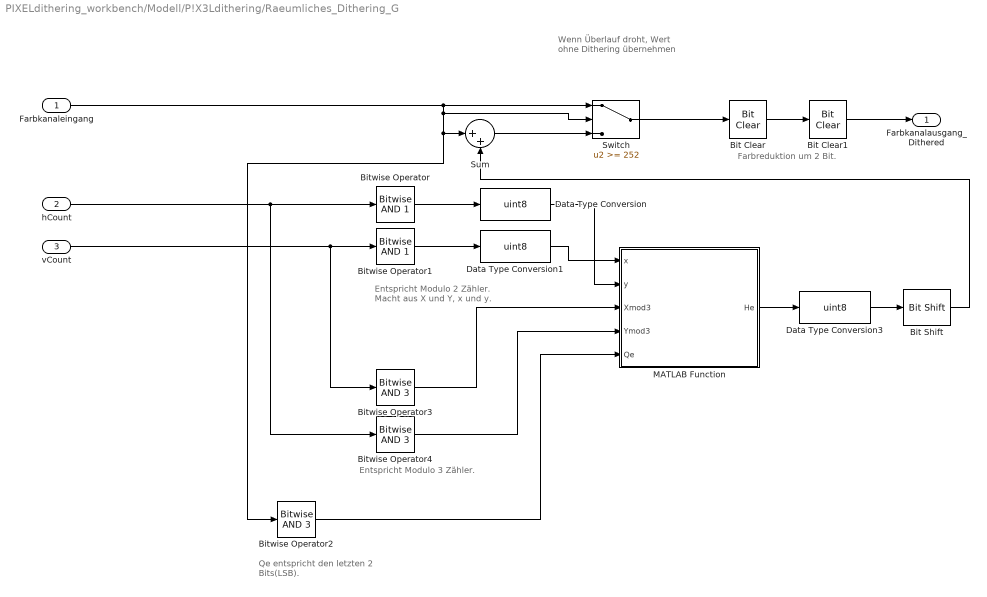
== system PIXELdithering_workbench/Modell/P!X3Ldithering/Raeumliches_Dithering_G ==
  note: Entspricht
      | Modulo 3 Zähler.
  note: Qe entspricht den
      | letzten 2 Bits(LSB).
  note: Wenn Überlauf droht,
      | Wert ohne Dithering
      | übernehmen
  note: Farbreduktion um 2 Bit.
  note: Entspricht
      | Modulo 2 Zähler.
      | Macht aus X und Y,
      | x und y.
  Farbkanaleingang : Inport
  hCount : Inport  Port=2
  vCount : Inport  Port=3
  Bit Clear : simulink/Logic and Bit Operations/Bit Clear  iBit=0
      settings: SourceProductBaseCode=SL
  Bit Clear1 : simulink/Logic and Bit Operations/Bit Clear  iBit=1
      settings: SourceProductBaseCode=SL
  Bit Shift : hdlsllib/Logic and Bit Operations/Bit Shift  mode=Shift Left Logical  N=2
  Bitwise Operator : simulink/Logic and Bit Operations/Bitwise Operator  logicop=AND  UseBitMask=on  BitMask=1  BitMaskRealWorld=Stored Integer
  Bitwise Operator1 : simulink/Logic and Bit Operations/Bitwise Operator  logicop=AND  UseBitMask=on  BitMask=1  BitMaskRealWorld=Stored Integer
  Bitwise Operator2 : simulink/Logic and Bit Operations/Bitwise Operator  logicop=AND  UseBitMask=on  BitMask=3  BitMaskRealWorld=Stored Integer
  Bitwise Operator3 : simulink/Logic and Bit Operations/Bitwise Operator  logicop=AND  UseBitMask=on  BitMask=3  BitMaskRealWorld=Stored Integer
  Bitwise Operator4 : simulink/Logic and Bit Operations/Bitwise Operator  logicop=AND  UseBitMask=on  BitMask=3  BitMaskRealWorld=Stored Integer
  Data Type Conversion : DataTypeConversion  OutDataTypeStr=uint8
  Data Type Conversion1 : DataTypeConversion  OutDataTypeStr=uint8
  Data Type Conversion3 : DataTypeConversion  OutDataTypeStr=uint8
  MATLAB Function : MATLAB Function  TreatAsAtomicUnit=on
  Sum : Sum  Inputs=|++
  Switch : Switch  Threshold=252
  Farbkanalausgang_Dithered : Outport
  wires:
  Farbkanaleingang/1 -> Switch/2, Bitwise Operator2/1, Sum/1, Switch/1
  Bit Clear/1 -> Bit Clear1/1
  Data Type Conversion1/1 -> MATLAB Function/1(x)
  hCount/1 -> Bitwise Operator4/1, Bitwise Operator/1
  Bitwise Operator1/1 -> Data Type Conversion1/1
  Bit Clear1/1 -> Farbkanalausgang_Dithered/1
  Data Type Conversion/1 -> MATLAB Function/2(y)
  vCount/1 -> Bitwise Operator3/1, Bitwise Operator1/1
  Bitwise Operator/1 -> Data Type Conversion/1
  Bit Shift/1 -> Sum/2
  Sum/1 -> Switch/3
  Switch/1 -> Bit Clear/1
  Data Type Conversion3/1 -> Bit Shift/1
  Bitwise Operator2/1 -> MATLAB Function/5(Qe)
  MATLAB Function/1(He) -> Data Type Conversion3/1
  Bitwise Operator3/1 -> MATLAB Function/3(Xmod3)
  Bitwise Operator4/1 -> MATLAB Function/4(Ymod3)

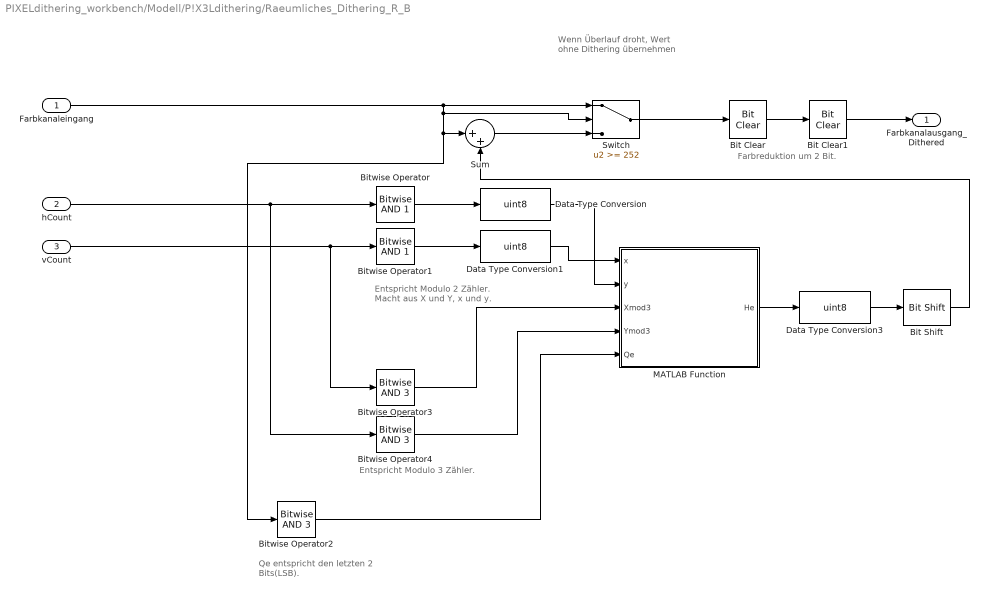
== system PIXELdithering_workbench/Modell/P!X3Ldithering/Raeumliches_Dithering_R_B ==
  note: Entspricht
      | Modulo 3 Zähler.
  note: Qe entspricht den
      | letzten 2 Bits(LSB).
  note: Wenn Überlauf droht,
      | Wert ohne Dithering
      | übernehmen
  note: Farbreduktion um 2 Bit.
  note: Entspricht
      | Modulo 2 Zähler.
      | Macht aus X und Y,
      | x und y.
  Farbkanaleingang : Inport
  hCount : Inport  Port=2
  vCount : Inport  Port=3
  Bit Clear : simulink/Logic and Bit Operations/Bit Clear  iBit=0
      settings: SourceProductBaseCode=SL
  Bit Clear1 : simulink/Logic and Bit Operations/Bit Clear  iBit=1
      settings: SourceProductBaseCode=SL
  Bit Shift : hdlsllib/Logic and Bit Operations/Bit Shift  mode=Shift Left Logical  N=2
  Bitwise Operator : simulink/Logic and Bit Operations/Bitwise Operator  logicop=AND  UseBitMask=on  BitMask=1  BitMaskRealWorld=Stored Integer
  Bitwise Operator1 : simulink/Logic and Bit Operations/Bitwise Operator  logicop=AND  UseBitMask=on  BitMask=1  BitMaskRealWorld=Stored Integer
  Bitwise Operator2 : simulink/Logic and Bit Operations/Bitwise Operator  logicop=AND  UseBitMask=on  BitMask=3  BitMaskRealWorld=Stored Integer
  Bitwise Operator3 : simulink/Logic and Bit Operations/Bitwise Operator  logicop=AND  UseBitMask=on  BitMask=3  BitMaskRealWorld=Stored Integer
  Bitwise Operator4 : simulink/Logic and Bit Operations/Bitwise Operator  logicop=AND  UseBitMask=on  BitMask=3  BitMaskRealWorld=Stored Integer
  Data Type Conversion : DataTypeConversion  OutDataTypeStr=uint8
  Data Type Conversion1 : DataTypeConversion  OutDataTypeStr=uint8
  Data Type Conversion3 : DataTypeConversion  OutDataTypeStr=uint8
  MATLAB Function : MATLAB Function  TreatAsAtomicUnit=on
  Sum : Sum  Inputs=|++
  Switch : Switch  Threshold=252
  Farbkanalausgang_Dithered : Outport
  wires:
  Farbkanaleingang/1 -> Switch/2, Bitwise Operator2/1, Sum/1, Switch/1
  Bit Clear/1 -> Bit Clear1/1
  Data Type Conversion1/1 -> MATLAB Function/1(x)
  hCount/1 -> Bitwise Operator4/1, Bitwise Operator/1
  Bitwise Operator1/1 -> Data Type Conversion1/1
  Bit Clear1/1 -> Farbkanalausgang_Dithered/1
  Data Type Conversion/1 -> MATLAB Function/2(y)
  vCount/1 -> Bitwise Operator3/1, Bitwise Operator1/1
  Bitwise Operator/1 -> Data Type Conversion/1
  Bit Shift/1 -> Sum/2
  Sum/1 -> Switch/3
  Switch/1 -> Bit Clear/1
  Data Type Conversion3/1 -> Bit Shift/1
  Bitwise Operator2/1 -> MATLAB Function/5(Qe)
  MATLAB Function/1(He) -> Data Type Conversion3/1
  Bitwise Operator3/1 -> MATLAB Function/3(Xmod3)
  Bitwise Operator4/1 -> MATLAB Function/4(Ymod3)

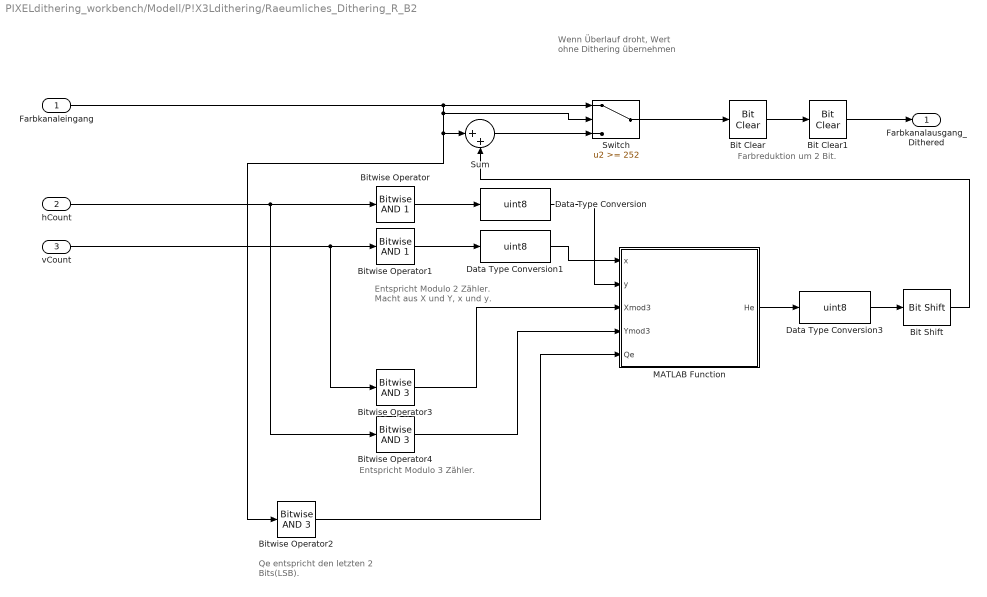
== system PIXELdithering_workbench/Modell/P!X3Ldithering/Raeumliches_Dithering_R_B2 ==
  note: Entspricht
      | Modulo 3 Zähler.
  note: Qe entspricht den
      | letzten 2 Bits(LSB).
  note: Wenn Überlauf droht,
      | Wert ohne Dithering
      | übernehmen
  note: Farbreduktion um 2 Bit.
  note: Entspricht
      | Modulo 2 Zähler.
      | Macht aus X und Y,
      | x und y.
  Farbkanaleingang : Inport
  hCount : Inport  Port=2
  vCount : Inport  Port=3
  Bit Clear : simulink/Logic and Bit Operations/Bit Clear  iBit=0
      settings: SourceProductBaseCode=SL
  Bit Clear1 : simulink/Logic and Bit Operations/Bit Clear  iBit=1
      settings: SourceProductBaseCode=SL
  Bit Shift : hdlsllib/Logic and Bit Operations/Bit Shift  mode=Shift Left Logical  N=2
  Bitwise Operator : simulink/Logic and Bit Operations/Bitwise Operator  logicop=AND  UseBitMask=on  BitMask=1  BitMaskRealWorld=Stored Integer
  Bitwise Operator1 : simulink/Logic and Bit Operations/Bitwise Operator  logicop=AND  UseBitMask=on  BitMask=1  BitMaskRealWorld=Stored Integer
  Bitwise Operator2 : simulink/Logic and Bit Operations/Bitwise Operator  logicop=AND  UseBitMask=on  BitMask=3  BitMaskRealWorld=Stored Integer
  Bitwise Operator3 : simulink/Logic and Bit Operations/Bitwise Operator  logicop=AND  UseBitMask=on  BitMask=3  BitMaskRealWorld=Stored Integer
  Bitwise Operator4 : simulink/Logic and Bit Operations/Bitwise Operator  logicop=AND  UseBitMask=on  BitMask=3  BitMaskRealWorld=Stored Integer
  Data Type Conversion : DataTypeConversion  OutDataTypeStr=uint8
  Data Type Conversion1 : DataTypeConversion  OutDataTypeStr=uint8
  Data Type Conversion3 : DataTypeConversion  OutDataTypeStr=uint8
  MATLAB Function : MATLAB Function  TreatAsAtomicUnit=on
  Sum : Sum  Inputs=|++
  Switch : Switch  Threshold=252
  Farbkanalausgang_Dithered : Outport
  wires:
  Farbkanaleingang/1 -> Switch/2, Bitwise Operator2/1, Sum/1, Switch/1
  Bit Clear/1 -> Bit Clear1/1
  Data Type Conversion1/1 -> MATLAB Function/1(x)
  hCount/1 -> Bitwise Operator4/1, Bitwise Operator/1
  Bitwise Operator1/1 -> Data Type Conversion1/1
  Bit Clear1/1 -> Farbkanalausgang_Dithered/1
  Data Type Conversion/1 -> MATLAB Function/2(y)
  vCount/1 -> Bitwise Operator3/1, Bitwise Operator1/1
  Bitwise Operator/1 -> Data Type Conversion/1
  Bit Shift/1 -> Sum/2
  Sum/1 -> Switch/3
  Switch/1 -> Bit Clear/1
  Data Type Conversion3/1 -> Bit Shift/1
  Bitwise Operator2/1 -> MATLAB Function/5(Qe)
  MATLAB Function/1(He) -> Data Type Conversion3/1
  Bitwise Operator3/1 -> MATLAB Function/3(Xmod3)
  Bitwise Operator4/1 -> MATLAB Function/4(Ymod3)

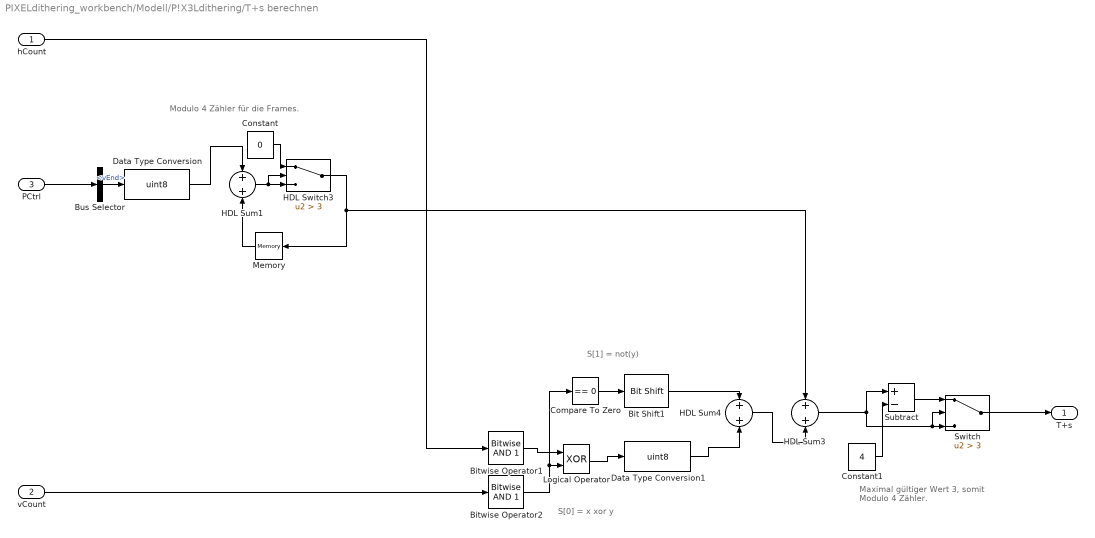
== system PIXELdithering_workbench/Modell/P!X3Ldithering/T+s berechnen ==
  note: Maximal gültiger Wert 3,
      | somit Modulo 4 Zähler.
  note: S[1] = not(y)
  note: S[0] = x xor y
  note: Modulo 4 Zähler für die Frames.
  hCount : Inport
  vCount : Inport  Port=2
  PCtrl : Inport  Port=3
  Bit Shift1 : hdlsllib/Logic and Bit Operations/Bit Shift  mode=Shift Left Logical  N=1
  Bitwise Operator1 : simulink/Logic and Bit Operations/Bitwise Operator  logicop=AND  UseBitMask=on  BitMask=1  BitMaskRealWorld=Stored Integer
  Bitwise Operator2 : simulink/Logic and Bit Operations/Bitwise Operator  logicop=AND  UseBitMask=on  BitMask=1  BitMaskRealWorld=Stored Integer
  Bus Selector : BusSelector  OutputSignals=vEnd
  Compare To Zero : simulink/Logic and Bit Operations/Compare To Zero  relop===  OutDataTypeStr=uint8
  Constant : Constant  Value=0  OutDataTypeStr=uint8  SampleTime=-1
  Constant1 : Constant  Value=4  OutDataTypeStr=uint8  SampleTime=-1
  Data Type Conversion : DataTypeConversion  OutMin=0  OutMax=1  OutDataTypeStr=uint8
  Data Type Conversion1 : DataTypeConversion  OutMin=0  OutMax=1  OutDataTypeStr=uint8
  HDL Sum1 : Sum  OutDataTypeStr=uint8  SaturateOnIntegerOverflow=on
  HDL Sum3 : Sum  OutDataTypeStr=uint8  SaturateOnIntegerOverflow=on
  HDL Sum4 : Sum  OutDataTypeStr=uint8  SaturateOnIntegerOverflow=on
  HDL Switch3 : Switch  Criteria=u2 > Threshold  Threshold=3  OutDataTypeStr=uint8
  Logical Operator : Logic  Operator=XOR  AllPortsSameDT=off  OutDataTypeStr=fixdt(1,16)
  Memory : Memory  InheritSampleTime=on
  Subtract : Sum  Inputs=+-
  Switch : Switch  Criteria=u2 > Threshold  Threshold=3
  T+s : Outport
  wires:
  Bit Shift1/1 -> HDL Sum4/1
  Bitwise Operator1/1 -> Logical Operator/1
  Compare To Zero/1 -> Bit Shift1/1
  Constant1/1 -> Subtract/2
  HDL Sum3/1 -> Switch/3, Switch/2, Subtract/1
  Subtract/1 -> Switch/1
  Data Type Conversion1/1 -> HDL Sum4/2
  Switch/1 -> T+s/1
  Logical Operator/1 -> Data Type Conversion1/1
  Bitwise Operator2/1 -> Compare To Zero/1, Logical Operator/2
  HDL Sum4/1 -> HDL Sum3/2
  HDL Switch3/1 -> HDL Sum3/1, Memory/1
  vCount/1 -> Bitwise Operator2/1
  hCount/1 -> Bitwise Operator1/1
  PCtrl/1 -> Bus Selector/1
  Bus Selector/1 -> Data Type Conversion/1  "<vEnd>"
  Memory/1 -> HDL Sum1/2
  HDL Sum1/1 -> HDL Switch3/2, HDL Switch3/3
  Constant/1 -> HDL Switch3/1
  Data Type Conversion/1 -> HDL Sum1/1

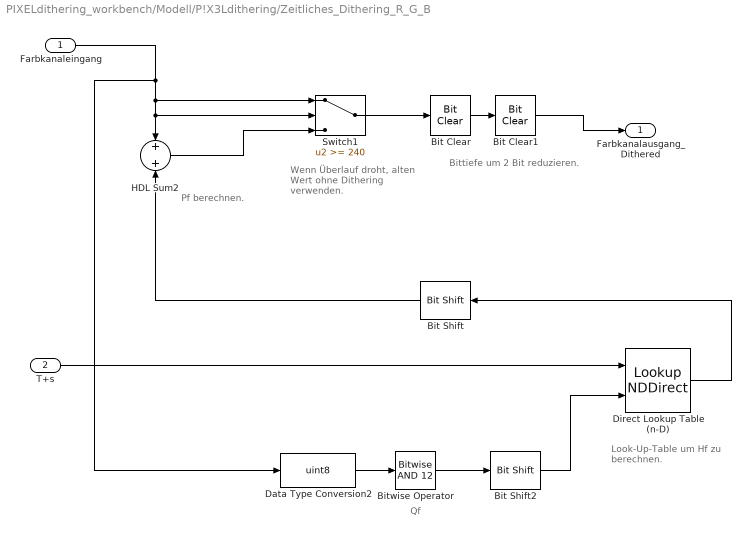
== system PIXELdithering_workbench/Modell/P!X3Ldithering/Zeitliches_Dithering_R_G_B ==
  note: Pf berechnen.
  note: Wenn Überlauf droht,
      | alten Wert ohne Dithering verwenden.
  note: Bittiefe um 2 Bit
      | reduzieren.
  note: Look-Up-Table um Hf
      | zu berechnen.
  note: Qf
  Farbkanaleingang : Inport
  T+s : Inport  Port=2
  Bit Clear : simulink/Logic and Bit Operations/Bit Clear  iBit=2
      settings: SourceProductBaseCode=SL
  Bit Clear1 : simulink/Logic and Bit Operations/Bit Clear  iBit=3
      settings: SourceProductBaseCode=SL
  Bit Shift : hdlsllib/Logic and Bit Operations/Bit Shift  mode=Shift Left Logical  N=4
  Bit Shift2 : hdlsllib/Logic and Bit Operations/Bit Shift  mode=Shift Right Logical  N=2
  Bitwise Operator : simulink/Logic and Bit Operations/Bitwise Operator  logicop=AND  UseBitMask=on  BitMask=12  BitMaskRealWorld=Stored Integer
  Data Type Conversion2 : DataTypeConversion  OutDataTypeStr=uint8
  Direct Lookup Table (n-D) : LookupNDDirect  Table=[0 1 1 0; 0 0 0 1; 0 0 1 1; 0 0 0 1]  DiagnosticForOutOfRangeInput=Error  TableDataTypeStr=uint8
  HDL Sum2 : Sum  OutDataTypeStr=uint8  SaturateOnIntegerOverflow=on
  Switch1 : Switch  Threshold=240
  Farbkanalausgang_Dithered : Outport
  wires:
  Direct Lookup Table (n-D)/1 -> Bit Shift/1
  Bit Shift/1 -> HDL Sum2/2
  Farbkanaleingang/1 -> Switch1/1, Switch1/2, HDL Sum2/1, Data Type Conversion2/1
  Bit Clear/1 -> Bit Clear1/1
  Bit Clear1/1 -> Farbkanalausgang_Dithered/1
  Bitwise Operator/1 -> Bit Shift2/1
  Bit Shift2/1 -> Direct Lookup Table (n-D)/2
  Data Type Conversion2/1 -> Bitwise Operator/1
  HDL Sum2/1 -> Switch1/3
  Switch1/1 -> Bit Clear/1
  T+s/1 -> Direct Lookup Table (n-D)/1
